simulink model "PID_Simulation_System_Paper"  (R2018b)
settings: Solver=VariableStepAuto  StartTime=0.0  StopTime=30  RelTol=1e-3
undefined symbols (not defined in the file): B, b, g, h, initial_theta, Jeq, Kb, kd, ki, Km, kp, l, La, M, m, N, r, Ra
libraries: simulink x1, simulink_extras x1
settings Model: Creator=fred  LastModifiedBy=fredericovaz
settings SolverCC: AlgebraicLoopSolver=LineSearch
settings HardwareCC: ProdBitPerLong=64  ProdHWDeviceType=Intel->x86-64 (Linux 64)

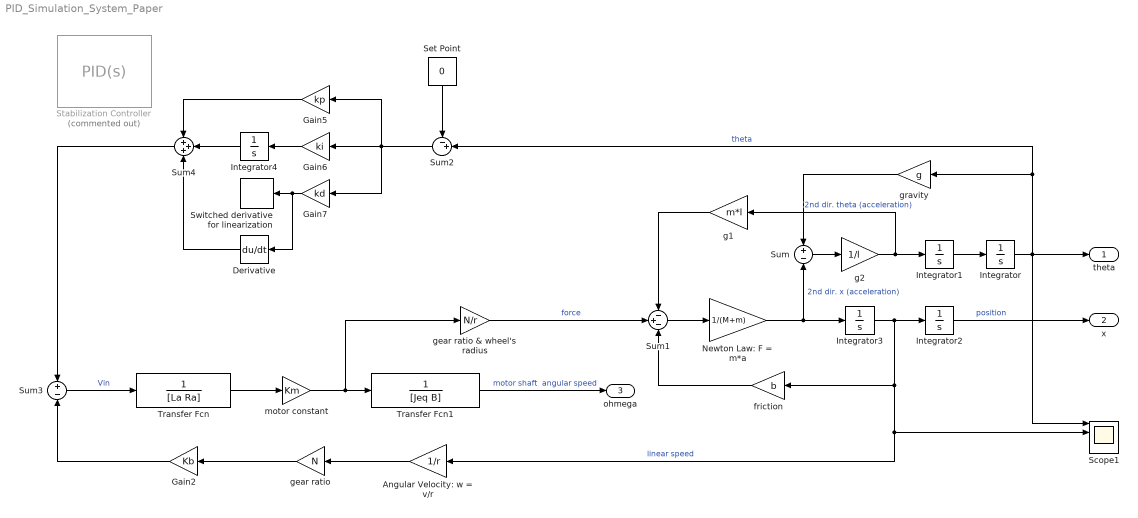
== system PID_Simulation_System_Paper ==
  Angular Velocity: w = v/r : Gain  Gain=1/r
  Derivative : Derivative
  Gain2 : Gain  Gain=Kb
  Gain5 : Gain  Gain=kp
  Gain6 : Gain  Gain=ki
  Gain7 : Gain  Gain=kd
  Integrator : Integrator  InitialCondition=initial_theta
  Integrator{1..4} (4 alike) : Integrator
  Newton Law: F = m*a : Gain  Gain=1/(M+m)
  Scope1 : Scope  NumInputPorts=4
  Set Point : Constant  Value=0
  Stabilization Controller : simulink/Continuous/PID Controller  Commented=on  Controller=PID  Form=Parallel  TimeDomain=Continuous-time  SampleTime=h  IntegratorMethod=Forward Euler  FilterMethod=Forward Euler  ControllerParametersSource=internal  P=4000  I=50  D=1200  UseFilter=on  N=50  TunerSelectOption=Transfer Function Based (PID Tuner App)  InitialConditionSource=internal  InitialConditionForIntegrator=0  InitialConditionForFilter=0  DifferentiatorICPrevScaledInput=0  ExternalReset=none  TrackingMode=off  Kt=1  LimitOutput=off  UpperSaturationLimit=inf  LowerSaturationLimit=-inf  LinearizeAsGain=on  AntiWindupMode=none  Kb=1  POutMin=[]  POutMax=[]  IOutMin=[]  IOutMax=[]  DOutMin=[]  DOutMax=[]  NOutMin=[]  NOutMax=[]  SumOutMin=[]  SumOutMax=[]  SaturationOutMin=[]  SaturationOutMax=[]  PParamMin=[]  PParamMax=[]  IParamMin=[]  IParamMax=[]  DParamMin=[]  DParamMax=[]  NParamMin=[]  NParamMax=[]  KbParamMin=[]  KbParamMax=[]  KtParamMin=[]  KtParamMax=[]  KbOutMin=[]  KbOutMax=[]  KtOutMin=[]  KtOutMax=[]  IntegratorOutMin=[]  IntegratorOutMax=[]  FilterOutMin=[]  FilterOutMax=[]  SumI1OutMin=[]  SumI1OutMax=[]  SumI2OutMin=[]  SumI2OutMax=[]  SumI3OutMin=[]  SumI3OutMax=[]  SumI4OutMin=[]  SumI4OutMax=[]  SumDOutMin=[]  SumDOutMax=[]  DifferentiatorOutMin=[]  DifferentiatorOutMax=[]  FilterDiffOutCoefMin=[]  FilterDiffOutCoefMax=[]  ReciprocalOutMin=[]  ReciprocalOutMax=[]  SumDenOutMin=[]  SumDenOutMax=[]  SumNumOutMin=[]  SumNumOutMax=[]  DivideOutMin=[]  DivideOutMax=[]  IntegratorContinuousStateAttributes=''  IntegratorStateMustResolveToSignalObject=off  IntegratorRTWStateStorageClass=Auto  FilterContinuousStateAttributes=''  FilterStateMustResolveToSignalObject=off  FilterRTWStateStorageClass=Auto  ParallelPVariant=InternalParameters  IdealPVariant=Disabled  IVariant=InternalParameters  DVariant=InternalParameters  IntegratorVariant=Continuous  SatVariant=Disabled  AWVariant=Passthrough  PCopyVariant=Disabled  TRVariant=Disabled  FdbkBlocksVariant=Forward  IdealPFdbkVariant=Disabled  SatFdbkVariant=Disabled  DerivativeFilterVariant=ContFilter  NVariant=InternalParameters  NCopyVariant=Disabled  FilterICVariant=InternalICsFilter  IntegratorICVariant=InternalICs  ExternalResetVariant=Disabled  TRSumVariant=Passthrough  SumFdbkVariant=Disabled  SumVariant=Sum_PID
  Sum : Sum  Inputs=+-
  Sum1 : Sum  Inputs=-+-
  Sum2 : Sum  Inputs=-+|
  Sum3 : Sum  Inputs=+-
  Sum4 : Sum  Inputs=+++
  Switched derivative for linearization : simulink_extras/Linearization/Switched derivative for linearization  switchVal=0  derivConst=100
      settings: SourceProductName=Simulink  SourceProductBaseCode=SL
  Transfer Fcn : TransferFcn  Denominator=[La Ra]
  Transfer Fcn1 : TransferFcn  Denominator=[Jeq B]
  friction : Gain  Gain=b
  g1 : Gain  Gain=m*l
  g2 : Gain  Gain=1/l
  gear ratio : Gain  Gain=N
  gear ratio & wheel's radius : Gain  Gain=N/r
  gravity : Gain  Gain=g
  motor constant : Gain  Gain=Km
  theta : Outport
  x : Outport  Port=2
  ohmega : Outport  Port=3
  wires:
  motor constant/1 -> gear ratio & wheel's radius/1, Transfer Fcn1/1
  Gain2/1 -> Sum3/2
  Integrator/1 -> Scope1/1, Sum2/2, gravity/1, theta/1  "theta"
  Integrator2/1 -> x/1  "position"
  friction/1 -> Sum1/3
  Sum3/1 -> Transfer Fcn/1  "Vin"
  Transfer Fcn1/1 -> ohmega/1  "motor shaft  angular speed"
  Sum/1 -> g2/1
  Newton Law: F = m*a/1 -> Sum/2, Integrator3/1  "2nd dir. x (acceleration)"
  Integrator1/1 -> Integrator/1
  Integrator3/1 -> Scope1/2, Angular Velocity: w = v/r/1, friction/1, Integrator2/1  "linear speed"
  Transfer Fcn/1 -> motor constant/1
  Sum1/1 -> Newton Law: F = m*a/1
  gear ratio/1 -> Gain2/1
  g2/1 -> g1/1, Integrator1/1  "2nd dir. theta (acceleration)"
  g1/1 -> Sum1/1
  gear ratio & wheel's radius/1 -> Sum1/2  "force"
  Angular Velocity: w = v/r/1 -> gear ratio/1
  gravity/1 -> Sum/1
  Set Point/1 -> Sum2/1
  Gain7/1 -> Derivative/1, Switched derivative for linearization/1
  Gain5/1 -> Sum4/1
  Gain6/1 -> Integrator4/1
  Integrator4/1 -> Sum4/2
  Sum2/1 -> Gain5/1, Gain7/1, Gain6/1
  Sum4/1 -> Sum3/1
  Derivative/1 -> Sum4/3
